simulink model "final_hover_final"  (R2019a)
settings: Solver=VariableStepAuto  StartTime=0.0  StopTime=inf  RelTol=1e-3
undefined symbols (not defined in the file): DiscIntNeverNeededParam
libraries: simulink x4, shared6dof x1, simulink_extras x1, slctrlblks x1, robotuavlib x1
settings Model: Creator=chait  LastModifiedBy=DINESH

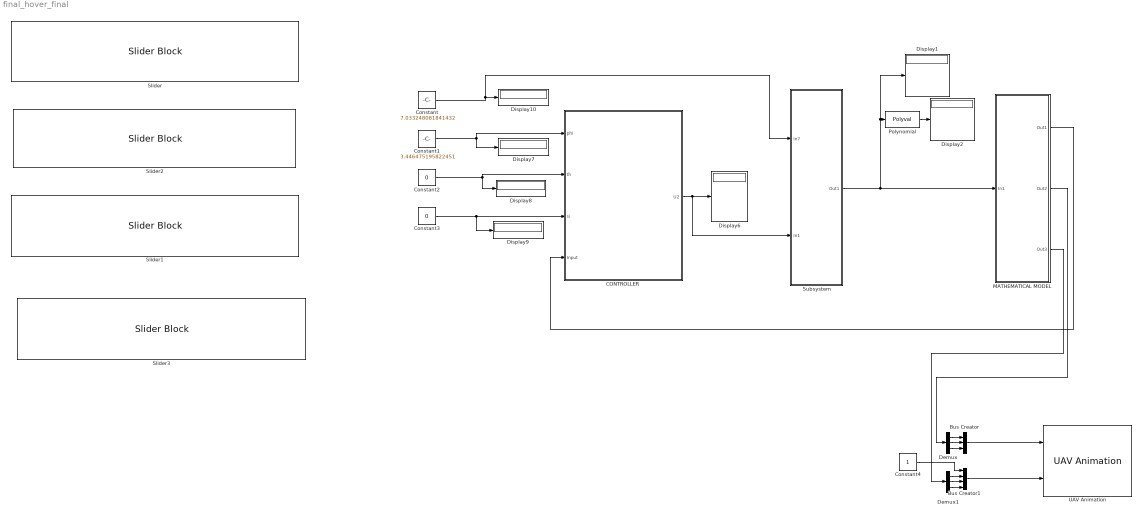
== system final_hover_final ==
  " MATHEMATICAL MODEL" : Subsystem
  Bus Creator : BusCreator  Inputs=3
  Bus Creator1 : BusCreator  Inputs=4
  CONTROLLER : Subsystem
  Constant : Constant  Value=7.033248081841432
  Constant1 : Constant  Value=3.446475195822451
  Constant2 : Constant  Value=0
  Constant3 : Constant  Value=0
  Constant4 : Constant
  Demux : Demux  Outputs=3
  Demux1 : Demux  Outputs=3
  Display{1..2,6..10} (7 alike) : Display
  Polynomial : Polyval  Coefs=[1.126e-05 0.05526 1000]
  Slider : SliderBlock  ScaleMax=20
  Slider1 : SliderBlock  ScaleMin=-30  ScaleMax=30
  Slider2 : SliderBlock  ScaleMin=-30  ScaleMax=30
  Slider3 : SliderBlock  ScaleMin=-30  ScaleMax=30
  Subsystem : Subsystem
  UAV Animation : robotuavlib/UAV Animation  UAVType=Multirotor  UAVSize=10  InertialZDirection=Up  SampleTime=-1
      settings: SourceProductName=Robotics System Toolbox UAV Library  SourceProductBaseCode=ROBOTICS_UAV_LIB
  wires:
  Constant2/1 -> CONTROLLER/2(th), Display8/1
  Constant/1 -> Subsystem/1(In7), Display10/1
  Constant1/1 -> CONTROLLER/1(phi), Display7/1
  Subsystem/1(Out1) -> " MATHEMATICAL MODEL"/1(In1), Display1/1, Polynomial/1
  " MATHEMATICAL MODEL"/1(Out1) -> CONTROLLER/4(Input)
  Polynomial/1 -> Display2/1
  CONTROLLER/1(U2) -> Subsystem/2(In1), Display6/1
  Constant3/1 -> Display9/1, CONTROLLER/3(si)
  Bus Creator1/1 -> UAV Animation/2
  Bus Creator/1 -> UAV Animation/1
  Demux/1 -> Bus Creator/1
  Demux/2 -> Bus Creator/2
  Demux/3 -> Bus Creator/3
  Demux1/3 -> Bus Creator1/4
  Demux1/2 -> Bus Creator1/3
  Demux1/1 -> Bus Creator1/2
  Constant4/1 -> Bus Creator1/1
  " MATHEMATICAL MODEL"/2(Out2) -> Demux/1
  " MATHEMATICAL MODEL"/3(Out3) -> Demux1/1

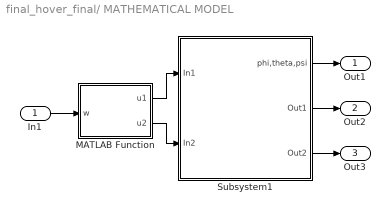
== system final_hover_final/ MATHEMATICAL MODEL ==
  In1 : Inport
  MATLAB Function : MATLAB Function  TreatAsAtomicUnit=on
  Subsystem1 : Subsystem
  Out1 : Outport
  Out2 : Outport  Port=2
  Out3 : Outport  Port=3
  wires:
  Subsystem1/1(phi,theta,psi) -> Out1/1
  MATLAB Function/1(u1) -> Subsystem1/1(In1)
  MATLAB Function/2(u2) -> Subsystem1/2(In2)
  In1/1 -> MATLAB Function/1(w)
  Subsystem1/3(Out2) -> Out3/1
  Subsystem1/2(Out1) -> Out2/1

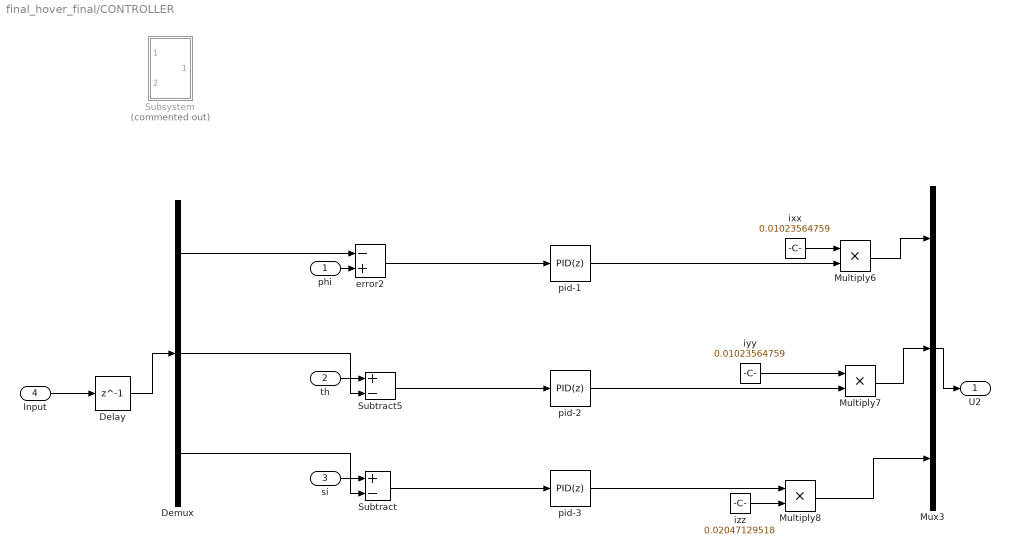
== system final_hover_final/CONTROLLER ==
  phi : Inport
  th : Inport  Port=2
  si : Inport  Port=3
  Input : Inport  Port=4
  Delay : Delay  DelayLength=1  SampleTime=0.04
  Demux : Demux  Outputs=3
  Multiply6 : Product  OutDataTypeStr=double
  Multiply7 : Product  OutDataTypeStr=double
  Multiply8 : Product  OutDataTypeStr=double
  Mux3 : Mux  Inputs=3
  Subsystem : Subsystem  Commented=on
  Subtract : Sum  Inputs=+-
  Subtract5 : Sum  Inputs=+-
  error2 : Sum  Inputs=-+
  ixx : Constant  Value=0.01023564759
  iyy : Constant  Value=0.01023564759
  izz : Constant  Value=0.02047129518
  pid-1 : simulink/Continuous/PID Controller  Controller=PID  Form=Parallel  TimeDomain=Discrete-time  SampleTime=-1  IntegratorMethod=Forward Euler  FilterMethod=Forward Euler  ControllerParametersSource=internal  P=8272.35058975293  I=302.479932874962  D=21767.3278850194  UseFilter=on  N=40.4121112016122  TunerSelectOption=Transfer Function Based (PID Tuner App)  InitialConditionSource=internal  InitialConditionForIntegrator=0  InitialConditionForFilter=0  DifferentiatorICPrevScaledInput=0  ExternalReset=none  TrackingMode=off  Kt=1  LimitOutput=off  UpperSaturationLimit=inf  LowerSaturationLimit=-inf  LinearizeAsGain=off  AntiWindupMode=none  Kb=1  POutMin=[]  POutMax=[]  IOutMin=[]  IOutMax=[]  DOutMin=[]  DOutMax=[]  NOutMin=[]  NOutMax=[]  SumOutMin=[]  SumOutMax=[]  SaturationOutMin=[]  SaturationOutMax=[]  PParamMin=[]  PParamMax=[]  IParamMin=[]  IParamMax=[]  DParamMin=[]  DParamMax=[]  NParamMin=[]  NParamMax=[]  KbParamMin=[]  KbParamMax=[]  KtParamMin=[]  KtParamMax=[]  KbOutMin=[]  KbOutMax=[]  KtOutMin=[]  KtOutMax=[]  IntegratorOutMin=[]  IntegratorOutMax=[]  FilterOutMin=[]  FilterOutMax=[]  SumI1OutMin=[]  SumI1OutMax=[]  SumI2OutMin=[]  SumI2OutMax=[]  SumI3OutMin=[]  SumI3OutMax=[]  SumI4OutMin=[]  SumI4OutMax=[]  SumDOutMin=[]  SumDOutMax=[]  DifferentiatorOutMin=[]  DifferentiatorOutMax=[]  FilterDiffOutCoefMin=[]  FilterDiffOutCoefMax=[]  ReciprocalOutMin=[]  ReciprocalOutMax=[]  SumDenOutMin=[]  SumDenOutMax=[]  SumNumOutMin=[]  SumNumOutMax=[]  DivideOutMin=[]  DivideOutMax=[]  IntegratorContinuousStateAttributes=''  IntegratorStateMustResolveToSignalObject=off  IntegratorRTWStateStorageClass=Auto  FilterContinuousStateAttributes=''  FilterStateMustResolveToSignalObject=off  FilterRTWStateStorageClass=Auto  ParallelPVariant=InternalParameters  IdealPVariant=Disabled  IVariant=InternalParameters  DVariant=InternalParameters  IntegratorVariant=Discrete  SatVariant=Disabled  AWVariant=Passthrough  PCopyVariant=Disabled  TRVariant=Disabled  FdbkBlocksVariant=Forward  IdealPFdbkVariant=Disabled  SatFdbkVariant=Disabled  DerivativeFilterVariant=ForwardEulerFilter  NVariant=InternalParameters  NCopyVariant=Disabled  FilterICVariant=InternalICsFilter  IntegratorICVariant=InternalICs  ExternalResetVariant=Disabled  TRSumVariant=Passthrough  SumFdbkVariant=Disabled  SumVariant=Sum_PID
  pid-2 : simulink/Continuous/PID Controller  Controller=PID  Form=Parallel  TimeDomain=Discrete-time  SampleTime=-1  IntegratorMethod=Forward Euler  FilterMethod=Forward Euler  ControllerParametersSource=internal  P=35610.9208208117  I=772.682830612308  D=364341.887091651  UseFilter=on  N=44.7394153654691  TunerSelectOption=Transfer Function Based (PID Tuner App)  InitialConditionSource=internal  InitialConditionForIntegrator=0  InitialConditionForFilter=0  DifferentiatorICPrevScaledInput=0  ExternalReset=none  TrackingMode=off  Kt=1  LimitOutput=off  UpperSaturationLimit=inf  LowerSaturationLimit=-inf  LinearizeAsGain=off  AntiWindupMode=none  Kb=1  POutMin=[]  POutMax=[]  IOutMin=[]  IOutMax=[]  DOutMin=[]  DOutMax=[]  NOutMin=[]  NOutMax=[]  SumOutMin=[]  SumOutMax=[]  SaturationOutMin=[]  SaturationOutMax=[]  PParamMin=[]  PParamMax=[]  IParamMin=[]  IParamMax=[]  DParamMin=[]  DParamMax=[]  NParamMin=[]  NParamMax=[]  KbParamMin=[]  KbParamMax=[]  KtParamMin=[]  KtParamMax=[]  KbOutMin=[]  KbOutMax=[]  KtOutMin=[]  KtOutMax=[]  IntegratorOutMin=[]  IntegratorOutMax=[]  FilterOutMin=[]  FilterOutMax=[]  SumI1OutMin=[]  SumI1OutMax=[]  SumI2OutMin=[]  SumI2OutMax=[]  SumI3OutMin=[]  SumI3OutMax=[]  SumI4OutMin=[]  SumI4OutMax=[]  SumDOutMin=[]  SumDOutMax=[]  DifferentiatorOutMin=[]  DifferentiatorOutMax=[]  FilterDiffOutCoefMin=[]  FilterDiffOutCoefMax=[]  ReciprocalOutMin=[]  ReciprocalOutMax=[]  SumDenOutMin=[]  SumDenOutMax=[]  SumNumOutMin=[]  SumNumOutMax=[]  DivideOutMin=[]  DivideOutMax=[]  IntegratorContinuousStateAttributes=''  IntegratorStateMustResolveToSignalObject=off  IntegratorRTWStateStorageClass=Auto  FilterContinuousStateAttributes=''  FilterStateMustResolveToSignalObject=off  FilterRTWStateStorageClass=Auto  ParallelPVariant=InternalParameters  IdealPVariant=Disabled  IVariant=InternalParameters  DVariant=InternalParameters  IntegratorVariant=Discrete  SatVariant=Disabled  AWVariant=Passthrough  PCopyVariant=Disabled  TRVariant=Disabled  FdbkBlocksVariant=Forward  IdealPFdbkVariant=Disabled  SatFdbkVariant=Disabled  DerivativeFilterVariant=ForwardEulerFilter  NVariant=InternalParameters  NCopyVariant=Disabled  FilterICVariant=InternalICsFilter  IntegratorICVariant=InternalICs  ExternalResetVariant=Disabled  TRSumVariant=Passthrough  SumFdbkVariant=Disabled  SumVariant=Sum_PID
  pid-3 : simulink/Continuous/PID Controller  Controller=PID  Form=Parallel  TimeDomain=Discrete-time  SampleTime=-1  IntegratorMethod=Forward Euler  FilterMethod=Forward Euler  ControllerParametersSource=internal  P=29.390290102355  I=0.436507766053145  D=439.41886339358  UseFilter=on  N=42.6692536316278  TunerSelectOption=Transfer Function Based (PID Tuner App)  InitialConditionSource=internal  InitialConditionForIntegrator=0  InitialConditionForFilter=0  DifferentiatorICPrevScaledInput=0  ExternalReset=none  TrackingMode=off  Kt=1  LimitOutput=off  UpperSaturationLimit=inf  LowerSaturationLimit=-inf  LinearizeAsGain=off  AntiWindupMode=none  Kb=1  POutMin=[]  POutMax=[]  IOutMin=[]  IOutMax=[]  DOutMin=[]  DOutMax=[]  NOutMin=[]  NOutMax=[]  SumOutMin=[]  SumOutMax=[]  SaturationOutMin=[]  SaturationOutMax=[]  PParamMin=[]  PParamMax=[]  IParamMin=[]  IParamMax=[]  DParamMin=[]  DParamMax=[]  NParamMin=[]  NParamMax=[]  KbParamMin=[]  KbParamMax=[]  KtParamMin=[]  KtParamMax=[]  KbOutMin=[]  KbOutMax=[]  KtOutMin=[]  KtOutMax=[]  IntegratorOutMin=[]  IntegratorOutMax=[]  FilterOutMin=[]  FilterOutMax=[]  SumI1OutMin=[]  SumI1OutMax=[]  SumI2OutMin=[]  SumI2OutMax=[]  SumI3OutMin=[]  SumI3OutMax=[]  SumI4OutMin=[]  SumI4OutMax=[]  SumDOutMin=[]  SumDOutMax=[]  DifferentiatorOutMin=[]  DifferentiatorOutMax=[]  FilterDiffOutCoefMin=[]  FilterDiffOutCoefMax=[]  ReciprocalOutMin=[]  ReciprocalOutMax=[]  SumDenOutMin=[]  SumDenOutMax=[]  SumNumOutMin=[]  SumNumOutMax=[]  DivideOutMin=[]  DivideOutMax=[]  IntegratorContinuousStateAttributes=''  IntegratorStateMustResolveToSignalObject=off  IntegratorRTWStateStorageClass=Auto  FilterContinuousStateAttributes=''  FilterStateMustResolveToSignalObject=off  FilterRTWStateStorageClass=Auto  ParallelPVariant=InternalParameters  IdealPVariant=Disabled  IVariant=InternalParameters  DVariant=InternalParameters  IntegratorVariant=Discrete  SatVariant=Disabled  AWVariant=Passthrough  PCopyVariant=Disabled  TRVariant=Disabled  FdbkBlocksVariant=Forward  IdealPFdbkVariant=Disabled  SatFdbkVariant=Disabled  DerivativeFilterVariant=ForwardEulerFilter  NVariant=InternalParameters  NCopyVariant=Disabled  FilterICVariant=InternalICsFilter  IntegratorICVariant=InternalICs  ExternalResetVariant=Disabled  TRSumVariant=Passthrough  SumFdbkVariant=Disabled  SumVariant=Sum_PID
  U2 : Outport
  wires:
  Mux3/1 -> U2/1
  izz/1 -> Multiply8/2
  ixx/1 -> Multiply6/1
  iyy/1 -> Multiply7/1
  Input/1 -> Delay/1
  Demux/2 -> Subtract5/2
  si/1 -> Subtract/1
  Demux/1 -> error2/1
  phi/1 -> error2/2
  Demux/3 -> Subtract/2
  th/1 -> Subtract5/1
  Delay/1 -> Demux/1
  pid-2/1 -> Multiply7/2
  Subtract5/1 -> pid-2/1
  pid-3/1 -> Multiply8/1
  Subtract/1 -> pid-3/1
  Multiply6/1 -> Mux3/1
  Multiply7/1 -> Mux3/2
  Multiply8/1 -> Mux3/3
  pid-1/1 -> Multiply6/2
  error2/1 -> pid-1/1

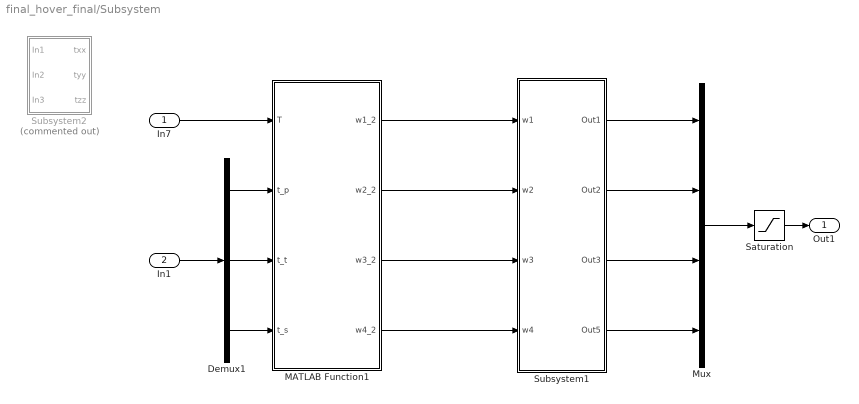
== system final_hover_final/Subsystem ==
  In7 : Inport
  In1 : Inport  Port=2
  Demux1 : Demux  Outputs=3
  MATLAB Function1 : MATLAB Function  TreatAsAtomicUnit=on
  Mux : Mux
  Saturation : Saturate  UpperLimit=7300  LowerLimit=0
  Subsystem1 : Subsystem
  Subsystem2 : Subsystem  Commented=on
  Out1 : Outport
  wires:
  Demux1/2 -> MATLAB Function1/3(t_t)
  Demux1/1 -> MATLAB Function1/2(t_p)
  Demux1/3 -> MATLAB Function1/4(t_s)
  In7/1 -> MATLAB Function1/1(T)
  MATLAB Function1/1(w1_2) -> Subsystem1/1(w1)
  MATLAB Function1/2(w2_2) -> Subsystem1/2(w2)
  MATLAB Function1/3(w3_2) -> Subsystem1/3(w3)
  MATLAB Function1/4(w4_2) -> Subsystem1/4(w4)
  In1/1 -> Demux1/1
  Subsystem1/4(Out5) -> Mux/4
  Subsystem1/1(Out1) -> Mux/1
  Subsystem1/3(Out3) -> Mux/3
  Subsystem1/2(Out2) -> Mux/2
  Saturation/1 -> Out1/1
  Mux/1 -> Saturation/1

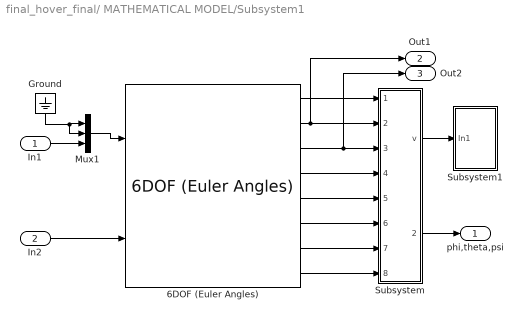
== system final_hover_final/ MATHEMATICAL MODEL/Subsystem1 ==
  In1 : Inport
  In2 : Inport  Port=2
  6DOF (Euler Angles) : shared6dof/6DOF (Euler Angles)  units=Metric (MKS)  mtype=Fixed  rep=Euler Angles  xme_0=[0 0 0]  Vm_0=[0 0 0]  eul_0=[0 0 0]  pm_0=[0 0 0]  mass_0=1.2  mass_e=0.5  mass_f=2.0  inertia=[0.01023564759,0,0;0,0.01023564759,0;0,0,0.02047129518]  inertia_e=eye(3)  inertia_f=2*eye(3)  k_quat=1.0  vre_flag=on  abi_flag=off  aMode=0  xme_statename=''  Vm_statename=''  eul_statename=''  quat_statename=''  pm_statename=''  mass_statename=''
      settings: SourceProductBaseCode=AE
  Ground : Ground
  Mux1 : Mux  Inputs=3
  Subsystem : Subsystem
  Subsystem1 : Subsystem
  phi,theta,psi : Outport
  Out1 : Outport  Port=2
  Out2 : Outport  Port=3
  wires:
  Ground/1 -> Mux1/2, Mux1/1
  Mux1/1 -> 6DOF (Euler Angles)/1
  In2/1 -> 6DOF (Euler Angles)/2
  In1/1 -> Mux1/3
  6DOF (Euler Angles)/1 -> Subsystem/1(In1)
  6DOF (Euler Angles)/2 -> Out1/1, Subsystem/2(In2)
  6DOF (Euler Angles)/3 -> Out2/1, Subsystem/3(In3)
  6DOF (Euler Angles)/4 -> Subsystem/4(In4)
  6DOF (Euler Angles)/5 -> Subsystem/5(In5)
  6DOF (Euler Angles)/6 -> Subsystem/6(In6)
  6DOF (Euler Angles)/7 -> Subsystem/7(In7)
  6DOF (Euler Angles)/8 -> Subsystem/8(In8)
  Subsystem/2(phi,theta,psi) -> phi,theta,psi/1
  Subsystem/1("v ") -> Subsystem1/1(In1)

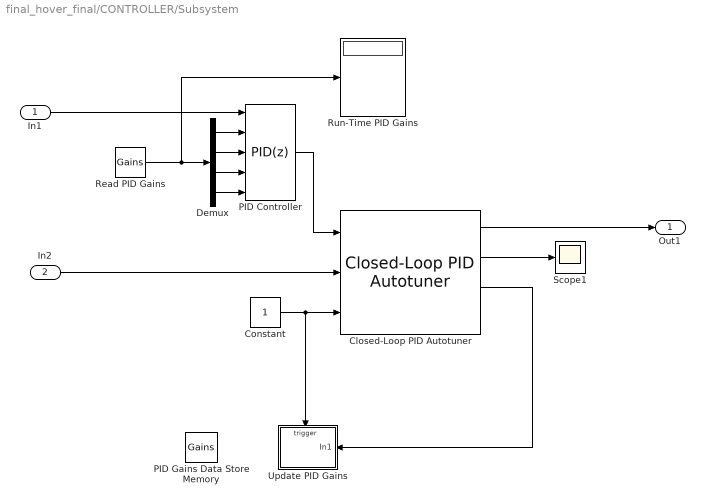
== system final_hover_final/CONTROLLER/Subsystem ==
  In1 : Inport
  In2 : Inport  Port=2
  Closed-Loop PID Autotuner : slctrlblks/Closed-Loop PID Autotuner  PIDType=PIDF  PIDForm=Parallel  TimeDomain=discrete-time  DiscreteTs=5e-6  IntegratorFormula=Forward Euler  FilterFormula=Forward Euler  ContinuousTs=0.02  Bandwidth=10000  UseExternalWC=off  TargetPM=60  UseExternalPM=off  UseExternalAchievedPM=off  PlantType=Stable  PlantSign=Positive  AmpSine=0.03  UseExternalAmpSine=off  UseExternalFRD=on  UseExternalU0=off  UseCompanion=off  NotDeployTuningModule=off  UsePLCCoder=off  OutputMode=control action + perturbation  BlockDataType=double  UseConnectedPID=on  blockpath=[]  tunedP=0  tunedI=0  tunedD=0  tunedN=100  tunedPM=0  EstimationWindowSize=3  OutputChoice=VariantCandD
      settings: SourceProductName=Simulink Control Design  SourceProductBaseCode=SD
  Constant : Constant
  Demux : Demux
  PID Controller : simulink/Continuous/PID Controller  Controller=PID  Form=Parallel  TimeDomain=Discrete-time  SampleTime=5e-6  IntegratorMethod=Forward Euler  FilterMethod=Forward Euler  ControllerParametersSource=external  P=0  I=140465083.2911  D=0  UseFilter=on  N=100  TunerSelectOption=Transfer Function Based (PID Tuner App)  InitialConditionSource=internal  InitialConditionForIntegrator=0  InitialConditionForFilter=0  DifferentiatorICPrevScaledInput=0  ExternalReset=none  TrackingMode=off  Kt=1  LimitOutput=on  UpperSaturationLimit=0.85  LowerSaturationLimit=0.1  LinearizeAsGain=on  AntiWindupMode=none  Kb=1  POutMin=[]  POutMax=[]  IOutMin=[]  IOutMax=[]  DOutMin=[]  DOutMax=[]  NOutMin=[]  NOutMax=[]  SumOutMin=[]  SumOutMax=[]  SaturationOutMin=[]  SaturationOutMax=[]  PParamMin=[]  PParamMax=[]  IParamMin=[]  IParamMax=[]  DParamMin=[]  DParamMax=[]  NParamMin=[]  NParamMax=[]  KbParamMin=[]  KbParamMax=[]  KtParamMin=[]  KtParamMax=[]  KbOutMin=[]  KbOutMax=[]  KtOutMin=[]  KtOutMax=[]  IntegratorOutMin=[]  IntegratorOutMax=[]  FilterOutMin=[]  FilterOutMax=[]  SumI1OutMin=[]  SumI1OutMax=[]  SumI2OutMin=[]  SumI2OutMax=[]  SumI3OutMin=[]  SumI3OutMax=[]  SumI4OutMin=[]  SumI4OutMax=[]  SumDOutMin=[]  SumDOutMax=[]  DifferentiatorOutMin=[]  DifferentiatorOutMax=[]  FilterDiffOutCoefMin=[]  FilterDiffOutCoefMax=[]  ReciprocalOutMin=[]  ReciprocalOutMax=[]  SumDenOutMin=[]  SumDenOutMax=[]  SumNumOutMin=[]  SumNumOutMax=[]  DivideOutMin=[]  DivideOutMax=[]  IntegratorContinuousStateAttributes=''  IntegratorStateMustResolveToSignalObject=off  IntegratorRTWStateStorageClass=Auto  FilterContinuousStateAttributes=''  FilterStateMustResolveToSignalObject=off  FilterRTWStateStorageClass=Auto  ParallelPVariant=ExternalParameters  IdealPVariant=Disabled  IVariant=ExternalParameters  DVariant=ExternalParameters  IntegratorVariant=Discrete  SatVariant=Enabled  AWVariant=Passthrough  PCopyVariant=Disabled  TRVariant=Disabled  FdbkBlocksVariant=Forward  IdealPFdbkVariant=Disabled  SatFdbkVariant=Disabled  DerivativeFilterVariant=ForwardEulerFilter  NVariant=ExternalParameters  NCopyVariant=Disabled  FilterICVariant=InternalICsFilter  IntegratorICVariant=InternalICs  ExternalResetVariant=Disabled  TRSumVariant=Passthrough  SumFdbkVariant=Disabled  SumVariant=Sum_PID
  PID Gains Data Store Memory : DataStoreMemory  DataStoreName=Gains  InitialValue=[0.02 160 5e-5 20000]  ShowAdditionalParam=off
  Read PID Gains : DataStoreRead  DataStoreName=Gains
  Run-Time PID Gains : Display
  Scope1 : Scope
  Update PID Gains : Subsystem
  Out1 : Outport
  wires:
  In1/1 -> PID Controller/1
  Read PID Gains/1 -> Run-Time PID Gains/1, Demux/1
  PID Controller/1 -> Closed-Loop PID Autotuner/1
  In2/1 -> Closed-Loop PID Autotuner/2
  Closed-Loop PID Autotuner/1 -> Out1/1
  Demux/1 -> PID Controller/2
  Closed-Loop PID Autotuner/3 -> Update PID Gains/1(In1)
  Constant/1 -> Closed-Loop PID Autotuner/3, Update PID Gains/Trigger
  Demux/3 -> PID Controller/4
  Closed-Loop PID Autotuner/2 -> Scope1/1
  Demux/2 -> PID Controller/3
  Demux/4 -> PID Controller/5

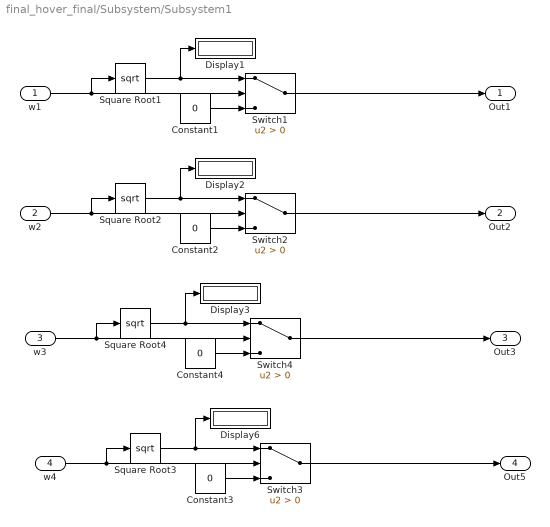
== system final_hover_final/Subsystem/Subsystem1 ==
  w1 : Inport
  w2 : Inport  Port=2
  w3 : Inport  Port=3
  w4 : Inport  Port=4
  Constant{1..4} (4 alike) : Constant  Value=0
  Display{1..3,6} (4 alike) : Display
  Square Root{1..4} (4 alike) : Sqrt  SaturateOnIntegerOverflow=on
  Switch{1..4} (4 alike) : Switch  Criteria=u2 > Threshold
  Out1 : Outport
  Out2 : Outport  Port=2
  Out3 : Outport  Port=3
  Out5 : Outport  Port=4
  wires:
  Square Root3/1 -> Switch3/1, Display6/1
  Constant3/1 -> Switch3/3
  w4/1 -> Switch3/2, Square Root3/1
  Switch3/1 -> Out5/1
  Square Root1/1 -> Switch1/1, Display1/1
  Switch1/1 -> Out1/1
  Constant1/1 -> Switch1/3
  w1/1 -> Switch1/2, Square Root1/1
  Square Root2/1 -> Switch2/1, Display2/1
  Switch2/1 -> Out2/1
  Constant2/1 -> Switch2/3
  w2/1 -> Switch2/2, Square Root2/1
  Square Root4/1 -> Switch4/1, Display3/1
  Switch4/1 -> Out3/1
  Constant4/1 -> Switch4/3
  w3/1 -> Switch4/2, Square Root4/1

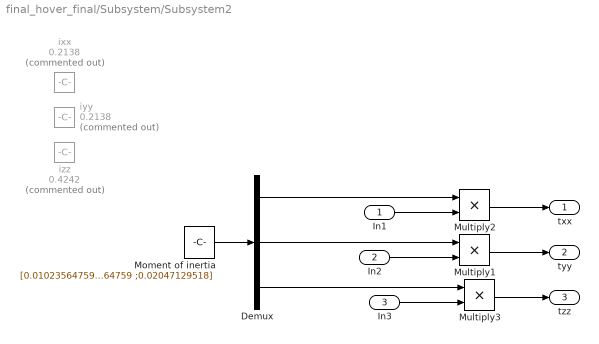
== system final_hover_final/Subsystem/Subsystem2 ==
  In1 : Inport
  In2 : Inport  Port=2
  In3 : Inport  Port=3
  Demux : Demux  Outputs=3
  Moment of inertia : Constant  Value=[0.01023564759 ;0.01023564759 ;0.02047129518]
  Multiply1 : Product  OutDataTypeStr=double
  Multiply2 : Product  OutDataTypeStr=double
  Multiply3 : Product  OutDataTypeStr=double
  ixx : Constant  Commented=on  Value=0.2138
  iyy : Constant  Commented=on  Value=0.2138
  izz : Constant  Commented=on  Value=0.4242
  txx : Outport
  tyy : Outport  Port=2
  tzz : Outport  Port=3
  wires:
  In1/1 -> Multiply2/2
  In3/1 -> Multiply3/2
  In2/1 -> Multiply1/2
  Demux/1 -> Multiply2/1
  Multiply2/1 -> txx/1
  Multiply1/1 -> tyy/1
  Multiply3/1 -> tzz/1
  Demux/3 -> Multiply3/1
  Demux/2 -> Multiply1/1
  Moment of inertia/1 -> Demux/1

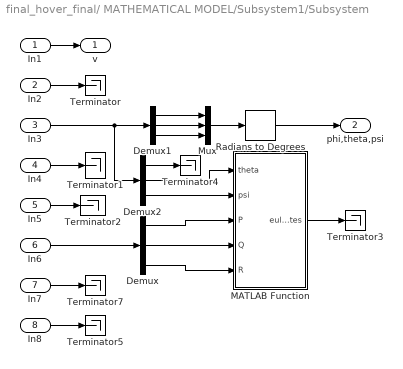
== system final_hover_final/ MATHEMATICAL MODEL/Subsystem1/Subsystem ==
  In1 : Inport
  In2 : Inport  Port=2
  In3 : Inport  Port=3
  In4 : Inport  Port=4
  In5 : Inport  Port=5
  In6 : Inport  Port=6
  In7 : Inport  Port=7
  In8 : Inport  Port=8
  Demux : Demux  Outputs=3
  Demux1 : Demux  Outputs=3
  Demux2 : Demux  Outputs=3
  MATLAB Function : MATLAB Function  TreatAsAtomicUnit=on
  Mux : Mux  Inputs=3
  Radians to Degrees : simulink_extras/Transformations/Radians to Degrees
  Terminator{,1..5,7} (7 alike) : Terminator
  "v " : Outport
  phi,theta,psi : Outport  Port=2
  wires:
  Demux1/1 -> Mux/1
  In3/1 -> Demux1/1, Demux2/1
  Demux2/1 -> Terminator4/1
  In1/1 -> "v "/1
  Mux/1 -> Radians to Degrees/1
  Demux1/2 -> Mux/2
  Demux1/3 -> Mux/3
  In8/1 -> Terminator5/1
  In4/1 -> Terminator1/1
  Demux/3 -> MATLAB Function/5(R)
  Demux2/2 -> MATLAB Function/1(theta)
  Demux/1 -> MATLAB Function/3(P)
  Demux2/3 -> MATLAB Function/2(psi)
  Demux/2 -> MATLAB Function/4(Q)
  In7/1 -> Terminator7/1
  In5/1 -> Terminator2/1
  In2/1 -> Terminator/1
  In6/1 -> Demux/1
  MATLAB Function/1(euler_rates) -> Terminator3/1
  Radians to Degrees/1 -> phi,theta,psi/1

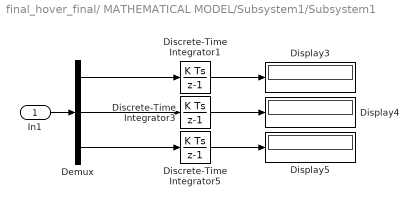
== system final_hover_final/ MATHEMATICAL MODEL/Subsystem1/Subsystem1 ==
  In1 : Inport
  Demux : Demux  Outputs=3
  Discrete-Time Integrator1 : DiscreteIntegrator  SampleTime=-1  ICPrevOutput=DiscIntNeverNeededParam  ICPrevScaledInput=DiscIntNeverNeededParam
  Discrete-Time Integrator3 : DiscreteIntegrator  SampleTime=-1  ICPrevOutput=DiscIntNeverNeededParam  ICPrevScaledInput=DiscIntNeverNeededParam
  Discrete-Time Integrator5 : DiscreteIntegrator  SampleTime=-1  ICPrevOutput=DiscIntNeverNeededParam  ICPrevScaledInput=DiscIntNeverNeededParam
  Display3 : Display
  Display4 : Display
  Display5 : Display
  wires:
  Demux/2 -> Discrete-Time Integrator3/1
  Demux/3 -> Discrete-Time Integrator5/1
  Discrete-Time Integrator3/1 -> Display4/1
  In1/1 -> Demux/1
  Discrete-Time Integrator5/1 -> Display5/1
  Discrete-Time Integrator1/1 -> Display3/1
  Demux/1 -> Discrete-Time Integrator1/1

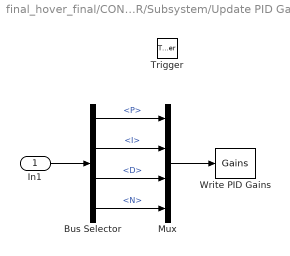
== system final_hover_final/CONTROLLER/Subsystem/Update PID Gains ==
  In1 : Inport
  Trigger : TriggerPort  TriggerType=falling  VariantControl=Variant  PortDimensions=1
  Bus Selector : BusSelector  OutputSignals=P,I,D,N
  Mux : Mux
  Write PID Gains : DataStoreWrite  DataStoreName=Gains
  wires:
  In1/1 -> Bus Selector/1
  Bus Selector/1 -> Mux/1  "<P>"
  Bus Selector/2 -> Mux/2  "<I>"
  Bus Selector/3 -> Mux/3  "<D>"
  Bus Selector/4 -> Mux/4  "<N>"
  Mux/1 -> Write PID Gains/1

== matlab function final_hover_final/ MATHEMATICAL MODEL/Subsystem1/Subsystem/MATLAB Function ==
  data: theta input; euler_rates output; psi input; P input; Q input; R input
function euler_rates = fcn(theta,psi,P,Q,R)

euler_rates = [(R.*cos(psi)+Q.*sin(psi))./cos(theta);
               Q.*cos(psi)-R.*sin(psi);
               (P.*cos(theta)+R.*cos(psi).*sin(theta)+Q.*sin(psi).*sin(theta))./cos(theta)];
end

== matlab function final_hover_final/Subsystem/MATLAB Function1 ==
  data: T input; t_p input; t_t input; t_s input; w1_2 output; w2_2 output; w3_2 output; w4_2 output
function [w1_2,w2_2,w3_2,w4_2] = fcn(T,t_p,t_t,t_s)
% ct = 8.586e-08;
% cq = 4.81e-09;
ct = 8.232*10^-8;
cq = 4.832*10^-9;
d  = 0.162635;%meters
 
 co = [ct ct ct ct;
      -d*ct d*ct d*ct -d*ct;
      -d*ct -d*ct d*ct d*ct;
      -cq cq -cq cq];
 i =  (inv(co));
 im = [T;t_p;t_t;t_s] ;
   w = i*im ; 

   w1_2 = w(1,1);
   w2_2 = w(2,1);
   w3_2 = w(3,1);
   w4_2 = w(4,1);
   
     
   
end

== matlab function final_hover_final/ MATHEMATICAL MODEL/MATLAB Function ==
  data: w input; u1 output; u2 output
function [u1,u2] = fcn(w)
ct = 8.586e-08;
cq = 4.81e-09;
d  = 0.176777;%meters
 
 co = [ct ct ct ct;
      -d*ct d*ct d*ct -d*ct;
      -d*ct -d*ct d*ct d*ct;
      -cq cq -cq cq];

  y = co*w;
  u1 = y(1);
  u2 = y(2:4);
end
